simulink model "diec_architecture_model"  (R2024a)
settings: Solver=VariableStepAuto  StartTime=0.0  StopTime=10.0  RelTol=1e-3
settings Model: Creator=prony  LastModifiedBy=prony

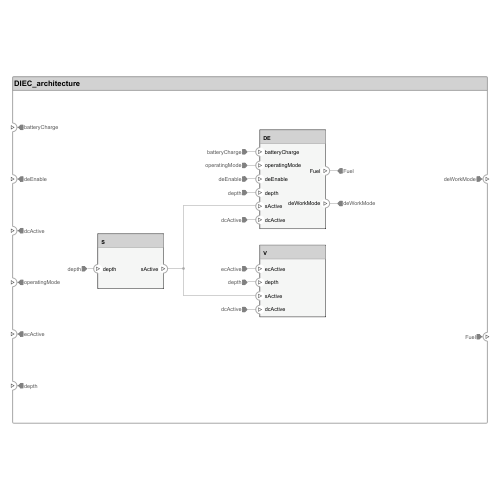
[thumbnail: Simulink's stored preview of the top-level diagram]
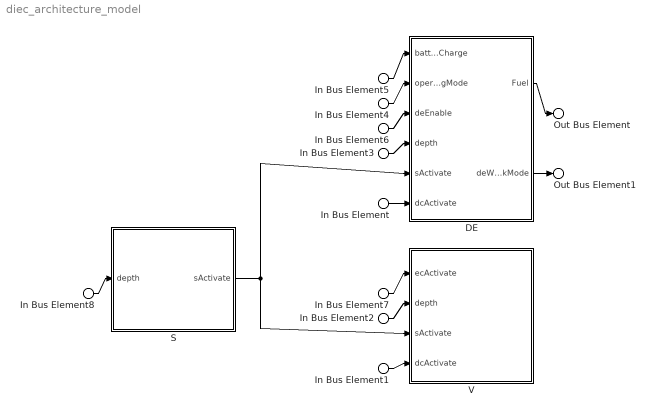
== system diec_architecture_model ==
  In Bus Element5 : Inport  PortName=batteryCharge
  In Bus Element6 : Inport  Port=2  PortName=deEnable
  In Bus Element : Inport  Port=3  PortName=dcActivate
  In Bus Element1 : Inport  Port=3  PortName=dcActivate
  In Bus Element4 : Inport  Port=4  PortName=operatingMode
  In Bus Element7 : Inport  Port=5  PortName=ecActivate
  In Bus Element2 : Inport  Port=6  PortName=depth
  In Bus Element3 : Inport  Port=6  PortName=depth
  In Bus Element8 : Inport  Port=6  PortName=depth
  DE : Subsystem
      settings: PortSchema="{\"entries\":[{\"content\":{\"headerSize\":26,\"margin\":15,\"minimumSpacing\":25,\"sides\":[{\"content\":{\"connectorIds\":[\"In1\",\"In2\",\"In3\",\"In4\",\"In5\",\"In6\"]},\"type\":\"ConnectorPlacement.EquallySpacedRectSide\",\"uuid\":\"a081745d-e304-460c-b260-28f873f47412\"},{\"content\":{\"connectorIds\":[\"Out1\",\"Out2\"],\"side\":\"RIGHT\"},\"type\":\"ConnectorPlacement.EquallySpacedRectSide\",\"uuid\":\"dcf4b9c6-2480-4b38-b126-f720e2fbbdee\"},{\"content\":{\"side\":\"TOP\"},\"type\":\"ConnectorPlacement.EquallySpacedRectSide\",\"uuid\":\"2e0fe9f6-2011-40a0-8ce7-eb682ac58ad9\"}]},\"type\":\"ConnectorPlacement.EquallySpacedConnector\",\"uuid\":\"7c124dc1-cb37-4efe-b068-79fa1ddc3523\"}],\"packageUris\":[\"http://schema.mathworks.com/mf0/Connector/R2020b\"],\"version\":\"1.0\"}"
  S : Subsystem
      settings: PortSchema="{\"entries\":[{\"content\":{\"headerSize\":26,\"margin\":15,\"minimumSpacing\":25,\"sides\":[{\"content\":{\"connectorIds\":[\"In1\"]},\"type\":\"ConnectorPlacement.EquallySpacedRectSide\",\"uuid\":\"a081745d-e304-460c-b260-28f873f47412\"},{\"content\":{\"connectorIds\":[\"Out1\"],\"side\":\"RIGHT\"},\"type\":\"ConnectorPlacement.EquallySpacedRectSide\",\"uuid\":\"dcf4b9c6-2480-4b38-b126-f720e2fbbdee\"},{\"content\":{\"side\":\"TOP\"},\"type\":\"ConnectorPlacement.EquallySpacedRectSide\",\"uuid\":\"2e0fe9f6-2011-40a0-8ce7-eb682ac58ad9\"}]},\"type\":\"ConnectorPlacement.EquallySpacedConnector\",\"uuid\":\"7c124dc1-cb37-4efe-b068-79fa1ddc3523\"}],\"packageUris\":[\"http://schema.mathworks.com/mf0/Connector/R2020b\"],\"version\":\"1.0\"}"
  V : Subsystem
      settings: PortSchema="{\"entries\":[{\"content\":{\"headerSize\":26,\"margin\":15,\"minimumSpacing\":25,\"sides\":[{\"content\":{\"connectorIds\":[\"In1\",\"In2\",\"In3\",\"In4\"]},\"type\":\"ConnectorPlacement.EquallySpacedRectSide\",\"uuid\":\"a081745d-e304-460c-b260-28f873f47412\"},{\"content\":{\"side\":\"RIGHT\"},\"type\":\"ConnectorPlacement.EquallySpacedRectSide\",\"uuid\":\"dcf4b9c6-2480-4b38-b126-f720e2fbbdee\"},{\"content\":{\"side\":\"TOP\"},\"type\":\"ConnectorPlacement.EquallySpacedRectSide\",\"uuid\":\"2e0fe9f6-2011-40a0-8ce7-eb682ac58ad9\"}]},\"type\":\"ConnectorPlacement.EquallySpacedConnector\",\"uuid\":\"7c124dc1-cb37-4efe-b068-79fa1ddc3523\"}],\"packageUris\":[\"http://schema.mathworks.com/mf0/Connector/R2020b\"],\"version\":\"1.0\"}"
  Out Bus Element1 : Outport  PortName=deWorkMode
  Out Bus Element : Outport  Port=2  PortName=Fuel
  wires:
  DE/1(Fuel) -> Out Bus Element/1
  DE/2(deWorkMode) -> Out Bus Element1/1
  S/1(sActivate) -> V/3(sActivate), DE/5(sActivate)
  In Bus Element/1 -> DE/6(dcActivate)
  In Bus Element1/1 -> V/4(dcActivate)
  In Bus Element2/1 -> V/2(depth)
  In Bus Element3/1 -> DE/4(depth)
  In Bus Element4/1 -> DE/2(operatingMode)
  In Bus Element5/1 -> DE/1(batteryCharge)
  In Bus Element6/1 -> DE/3(deEnable)
  In Bus Element7/1 -> V/1(ecActivate)
  In Bus Element8/1 -> S/1(depth)

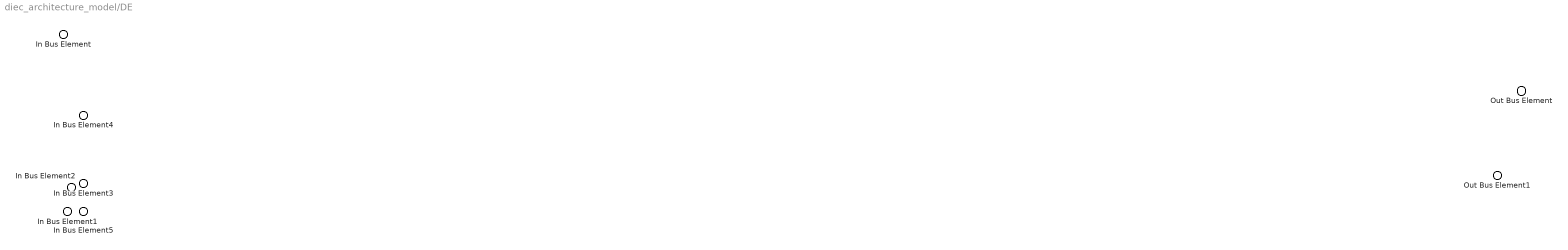
== system diec_architecture_model/DE ==
  In Bus Element1 : Inport  PortName=batteryCharge
  In Bus Element4 : Inport  Port=2  PortName=operatingMode
  In Bus Element5 : Inport  Port=3  PortName=deEnable
  In Bus Element3 : Inport  Port=4  PortName=depth
  In Bus Element2 : Inport  Port=5  PortName=sActivate
  In Bus Element : Inport  Port=6  PortName=dcActivate
  Out Bus Element1 : Outport  PortName=Fuel
  Out Bus Element : Outport  Port=2  PortName=deWorkMode

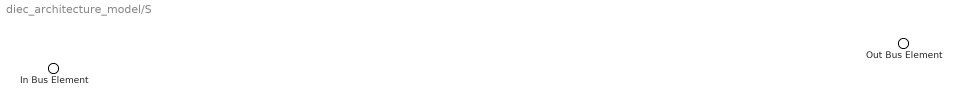
== system diec_architecture_model/S ==
  In Bus Element : Inport  PortName=depth
  Out Bus Element : Outport  PortName=sActivate

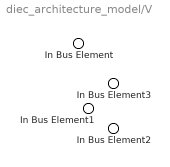
== system diec_architecture_model/V ==
  In Bus Element1 : Inport  PortName=ecActivate
  In Bus Element3 : Inport  Port=2  PortName=depth
  In Bus Element2 : Inport  Port=3  PortName=sActivate
  In Bus Element : Inport  Port=4  PortName=dcActivate
